simulink model "model_pt2_rl"  (R2020b)
settings: Solver=VariableStepAuto  StartTime=0.0  StopTime=5  RelTol=1e-3
undefined symbols (not defined in the file or in its folder): rl
libraries: rllib x1
settings Model: Creator=Julius  LastModifiedBy=Julius

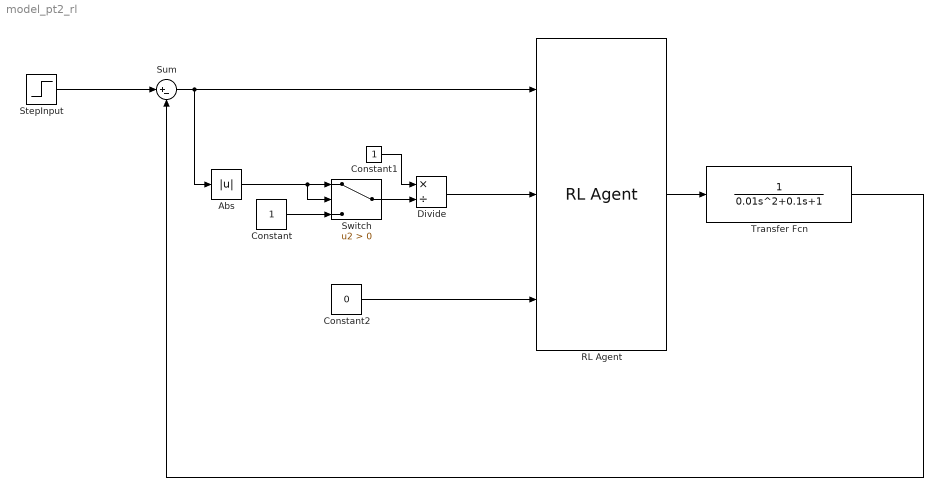
== system model_pt2_rl ==
  Abs : Abs
  Constant : Constant
  Constant1 : Constant
  Constant2 : Constant  Value=0
  Divide : Product  Inputs=*/
  RL Agent : rllib/RL Agent  Agent=rl.util.PolicyInstance.get('model_pt2_rl/RL Agent')  ProvideReward=on  ProvideIsDone=on  ProvideCumRwd=off  TreatAsDirectFeedthrough=on  CollectLoggedSignals=on  CollectModelStates=on
  StepInput : Step  SampleTime=0
  Sum : Sum  Inputs=|+-
  Switch : Switch  Criteria=u2 > Threshold
  Transfer Fcn : TransferFcn  Denominator=[0.01 0.1 1]
  wires:
  StepInput/1 -> Sum/1
  Transfer Fcn/1 -> Sum/2
  Sum/1 -> Abs/1, RL Agent/1
  Constant1/1 -> Divide/1
  Abs/1 -> Switch/1, Switch/2
  Constant2/1 -> RL Agent/3
  RL Agent/1 -> Transfer Fcn/1
  Switch/1 -> Divide/2
  Constant/1 -> Switch/3
  Divide/1 -> RL Agent/2
